simulink model "my_fuzzy2"  (R2023b)
settings: Solver=VariableStepAuto  StartTime=0.0  StopTime=16  RelTol=1e-3
libraries: fuzblock x1, SignalEditorBlockLib x1
settings Model: Creator=Αλέξανδρος Πετρίδης  LastModifiedBy=panospro
settings SolverCC: AlgebraicLoopSolver=TrustRegion
settings DebuggingCC: UnconnectedInputMsg=warning  UnconnectedOutputMsg=warning  UnconnectedLineMsg=warning
settings ModelReferenceCC: EnableRefExpFcnMdlSchedulingChecks=on

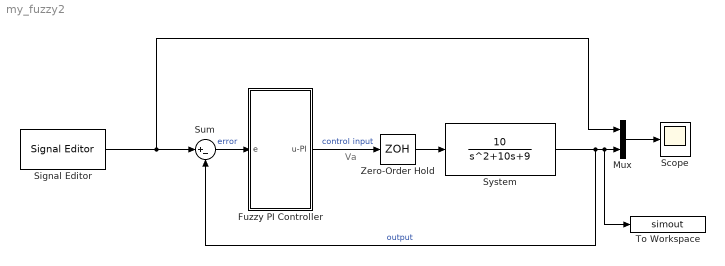
== system my_fuzzy2 ==
  note: Va
  Fuzzy PI Controller : Subsystem  TreatAsAtomicUnit=on
  Mux : Mux  Inputs=2
  Scope : Scope
  Signal Editor : SignalEditorBlockLib/Signal Editor  FileName=C:\Users\panospro\OneDrive\Υπολογιστής\Υπολογιστική 2023\Computational-Intelligence\Project 1\Scenario 2\graph 3.mat  ActiveScenario=Scenario  ActiveSignal=Signal  IsBus=off  OutputBusObjectStr=Bus: BusObject  SampleTime=0  Interpolate=off  ZeroCross=off  OutputAfterFinalValue=Setting to zero  Unit=inherit  PreserveSignalName=on  ApplySigPropsToAllScenarios=on  ApplySigPropsToAllSignals=off
  Sum : Sum  Inputs=|+-
  System : TransferFcn  Numerator=[10]  Denominator=[1 10 9]
  To Workspace : ToWorkspace  VariableName=simout  SaveFormat=Timeseries  SampleTime=-1
  Zero-Order Hold : ZeroOrderHold  SampleTime=-1
  wires:
  Sum/1 -> Fuzzy PI Controller/1(e)  "error"
  Fuzzy PI Controller/1(u-PI) -> Zero-Order Hold/1  "control input"
  Zero-Order Hold/1 -> System/1
  Mux/1 -> Scope/1
  Signal Editor/1 -> Mux/1, Sum/1
  System/1 -> To Workspace/1, Mux/2, Sum/2  "output"

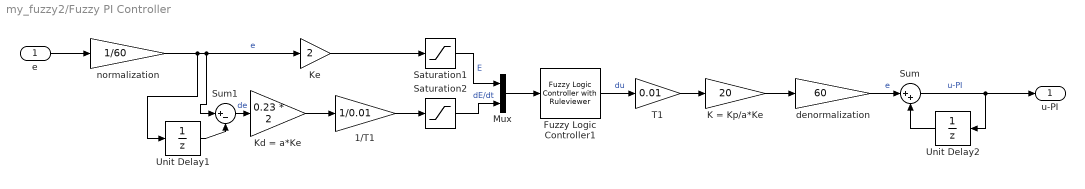
== system my_fuzzy2/Fuzzy PI Controller ==
  e : Inport
  1/T1 : Gain  Gain=1/0.01
  Fuzzy Logic Controller1 : fuzblock/Fuzzy Logic  Controller  with Ruleviewer  fismatrix=myfis  Ts=0.01
  "K = Kp/a*Ke " : Gain  Gain=20
  Kd = a*Ke : Gain  Gain=0.23 * 2
  Ke : Gain  Gain=2
  Mux : Mux  Inputs=2
  Saturation1 : Saturate  UpperLimit=1  LowerLimit=-1
  Saturation2 : Saturate  UpperLimit=1  LowerLimit=-1
  Sum : Sum  Inputs=|++
  Sum1 : Sum  Inputs=|+-
  T1 : Gain  Gain=0.01
  Unit Delay1 : UnitDelay  SampleTime=-1  HasFrameUpgradeWarning=on
  Unit Delay2 : UnitDelay  SampleTime=-1  HasFrameUpgradeWarning=on
  denormalization : Gain  Gain=60
  normalization : Gain  Gain=1/60
  u-PI : Outport
  wires:
  T1/1 -> "K = Kp/a*Ke "/1
  Sum/1 -> u-PI/1, Unit Delay2/1  "u-PI"
  Mux/1 -> Fuzzy Logic Controller1/1
  Kd = a*Ke/1 -> 1/T1/1
  normalization/1 -> Unit Delay1/1, Ke/1, Sum1/1  "e"
  Ke/1 -> Saturation1/1
  Sum1/1 -> Kd = a*Ke/1  "de"
  Unit Delay1/1 -> Sum1/2
  e/1 -> normalization/1
  1/T1/1 -> Saturation2/1
  Unit Delay2/1 -> Sum/2
  "K = Kp/a*Ke "/1 -> denormalization/1
  Fuzzy Logic Controller1/1 -> T1/1  "du"
  Saturation1/1 -> Mux/1  "E"
  Saturation2/1 -> Mux/2  "dE/dt"
  denormalization/1 -> Sum/1  "e"
